simulink subsystem "bTaskGrad"  (R2023a)
settings: Solver=VariableStepAuto  StartTime=0.0  StopTime=10.0  RelTol=1e-3
settings Model: Creator=KozlovM  LastModifiedBy=motya

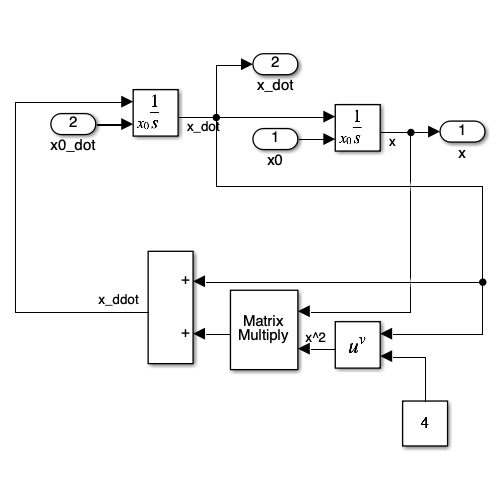
[thumbnail: Simulink's stored preview of the top-level diagram]
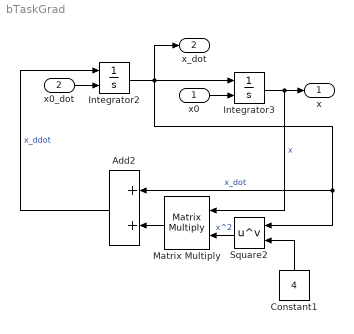
== system bTaskGrad ==
  x0 : Inport
  x0_dot : Inport  Port=2
  Add2 : Sum
  Constant1 : Constant  Value=4
  Integrator2 : Integrator  InitialConditionSource=external
  Integrator3 : Integrator  InitialConditionSource=external  InitialCondition=2
  Matrix Multiply : Product  Multiplication=Matrix(*)
  Square2 : Math  Operator=pow
  x : Outport
  x_dot : Outport  Port=2
  wires:
  Constant1/1 -> Square2/2
  x0_dot/1 -> Integrator2/2
  Add2/1 -> Integrator2/1  "x_ddot"
  x0/1 -> Integrator3/2
  Integrator2/1 -> x_dot/1, Integrator3/1, Add2/1, Square2/1  "x_dot"
  Integrator3/1 -> Matrix Multiply/1, x/1  "x"
  Square2/1 -> Matrix Multiply/2  "x^2"
  Matrix Multiply/1 -> Add2/2
